simulink model "AFTC"  (R2024a)
settings: Solver=VariableStepAuto  StartTime=0.0  StopTime=10.0  RelTol=1e-3
settings Model: Creator=Dell  LastModifiedBy=Dell

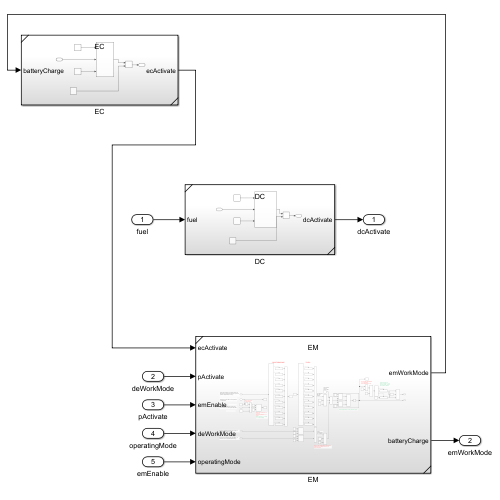
[thumbnail: Simulink's stored preview of the top-level diagram]
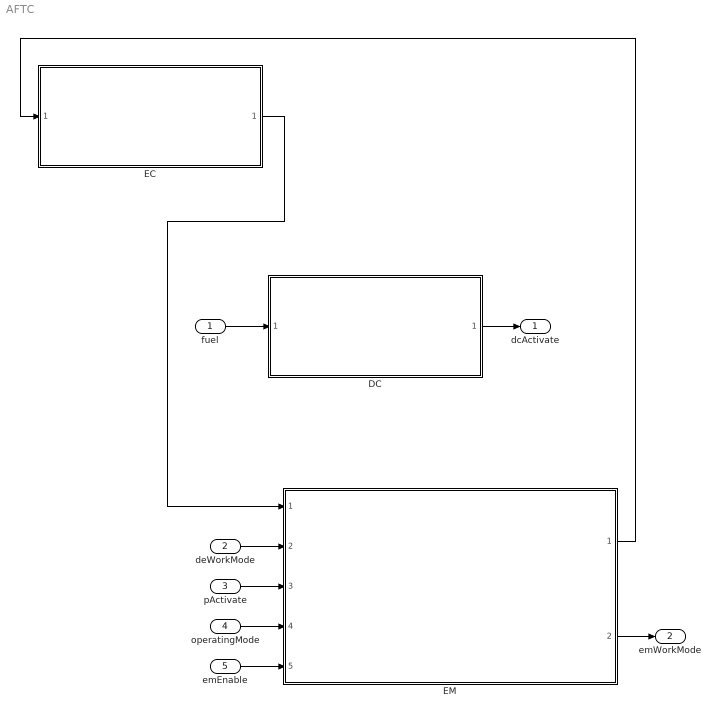
== system AFTC ==
  fuel : Inport
  deWorkMode : Inport  Port=2
  pActivate : Inport  Port=3
  operatingMode : Inport  Port=4
  emEnable : Inport  Port=5
  DC : Subsystem  ReferencedSubsystem=DC
  EC : Subsystem  ReferencedSubsystem=EC
  EM : Subsystem  ReferencedSubsystem=EM
  dcActivate : Outport
  emWorkMode : Outport  Port=2
  wires:
  EM/1 -> EC/1
  fuel/1 -> DC/1
  deWorkMode/1 -> EM/2
  EC/1 -> EM/1
  pActivate/1 -> EM/3
  operatingMode/1 -> EM/4
  emEnable/1 -> EM/5
  DC/1 -> dcActivate/1
  EM/2 -> emWorkMode/1
